simulink model "WindTurbine_System"  (R2023b)
settings: Solver=FixedStepAuto  StartTime=0.0  StopTime=24  FixedStep=1e-6  MaxStep=1e-6  RelTol=1e-3
values from neighbouring files (symbols this model uses):
  c1 = 0.22    [SystemParams.m]    (also in WindTurbineScript.m)
  c2 = 116    [SystemParams.m]    (also in WindTurbineScript.m)
  c3 = 0.4    [SystemParams.m]    (also in WindTurbineScript.m)
  c5 = 5    [SystemParams.m]    (also in WindTurbineScript.m)
  c6 = 12.5    [SystemParams.m]    (also in WindTurbineScript.m)
  C_boost = 50e-6    (= 5e-05)    [SystemParams.m]
  C_buck = 5e-6    (= 5e-06)    [SystemParams.m]
  C_rectifier = 1e-3    (= 0.001)    [SystemParams.m]
  Cp_sys = (Nr_cells_parallel * Cp_cell) / Nr_cells_series    [SystemParams.m]    (also in baterie.m)
  J = 0.8e-3    (= 0.0008)    [SystemParams.m]
  Ke = 0.175    [SystemParams.m]
  L_boost = 200e-6    (= 0.0002)    [SystemParams.m]
  L_buck = 300e-6    (= 0.0003)    [SystemParams.m]
  lambda_opt = 6.33    [SystemParams.m]    (also in WindTurbineScript.m)
  Ld = 1.53e-3    (= 0.00153)    [SystemParams.m]
  Lq = 1.53e-3    (= 0.00153)    [SystemParams.m]
  n1 = 15    [SystemParams.m]
  n2 = 1000    [SystemParams.m]
  omega_r = lambda_opt * wind_speed / R    (= 15.192)    [SystemParams.m]    (also in WindTurbineScript.m = omega_r_values(i))
  p = 4    [SystemParams.m]
  P_buck_v = 1.0e+03 * [0.01, 0.0427, 0.0854, 0.1282, 0.1709, 0.2136, 0.2563, 0.2990, 0.3418, 0.3845, 0.4272,                        0.4699, 0.5126, 0.5554, 0.5981, 0.6408, 0.6835, 0.7262, 0.7690, 0.8117, 0.8544,                        0.8971, 0.9398, 0.9826, 1.0253, 1.0680, 1.1107, 1.1534, 1.1962, 1.2389, 1.2816,                        1.3243, 1.3670, 1.4098, 1.4525, 1.4952, 1.5379, 1.5806, 1.6234, 1.6661, 1. ...(+623 chars)    [SystemParams.m]
  P_rec_v = 1.0e+03 * [0.01, 0.0432, 0.0864, 0.1296, 0.1727, 0.2159, 0.2591, 0.3023, 0.3455, 0.3887, 0.4319,                      0.4750, 0.5182, 0.5614, 0.6046, 0.6478, 0.6910, 0.7342, 0.7773, 0.8205, 0.8637,                      0.9069, 0.9501, 0.9933, 1.0365, 1.0796, 1.1228, 1.1660, 1.2092, 1.2524, 1.2956,                      1.3388, 1.3820, 1.4251, 1.4683, 1.5115, 1.5547, 1.5979, 1.6411, 1.6843, 1.7274,  ...(+605 chars)    [SystemParams.m]
  R = 5    [SystemParams.m]    (also in WindTurbineScript.m)
  R_buck_load_v = [230.4000, 53.9326, 26.9663, 17.9775, 13.4831, 10.7865, 8.9888, 7.7047, 6.7416, 5.9925, 5.3933,                   4.9030, 4.4944, 4.1487, 3.8523, 3.5955, 3.3708, 3.1725, 2.9963, 2.8386, 2.6966, 2.5682,                   2.4515, 2.3449, 2.2472, 2.1573, 2.0743, 1.9975, 1.9262, 1.8597, 1.7978, 1.7398, 1.6854,                   1.6343, 1.5863, 1.5409, 1.4981, 1.4576, 1.4193, 1.3829, 1.3483, 1.3154, 1. ...(+577 chars)    [SystemParams.m]
  R_rec_load_v = 1.0e+03 * [4.8400, 1.1204, 0.5602, 0.3735, 0.2803, 0.2242, 0.1868, 0.1601, 0.1401, 0.1245, 0.1121,                            0.1019, 0.0934, 0.0862, 0.0801, 0.0747, 0.0700, 0.0659, 0.0623, 0.0590, 0.0560, 0.0534,                            0.0509, 0.0487, 0.0467, 0.0448, 0.0431, 0.0415, 0.0400, 0.0386, 0.0374, 0.0362, 0.0350,                            0.0340, 0.0330, 0.0320, 0.0311, 0.0303, 0.02 ...(+634 chars)    [SystemParams.m]
  ro = 1.225    [SystemParams.m]    (also in WindTurbineScript.m)
  Rp_sys = (Nr_cells_series * Rp_cell) / Nr_cells_parallel    [SystemParams.m]    (also in baterie.m)
  Rs = 2.875    [SystemParams.m]    (also in VOC_1C_3pulse_14rest.mat = 0.09415625)
  Rs_sys = (Nr_cells_series * Rs_cell) / Nr_cells_parallel    [SystemParams.m]    (also in baterie.m)
  State_Of_Charge = 65    [SystemParams.m]
libraries: simulink x4, slpidlib x2, SignalEditorBlockLib x1
(part 2 of 2)

== stateflow chart WindTurbine_System/System Control ==
  state No_Wind_Power
    state Battery_Discharge
      entry, during:
      Boost_Control = 1;
      Battery_Control = 1;
      exit:
      Boost_Control = 0;
      Battery_Control = 0;
    state System_Off
      entry, during:
      Battery_Control = 1;
      Boost_Control = 0;
      Buck_Control = 0;
      WindTurbine_Control = 0;
    state Battery_Maintanance
      entry, during:
      Battery_Control = 0;
      Boost_Control = 0;
    (default) -> No_Wind_Power.System_Off
    No_Wind_Power.System_Off -> No_Wind_Power.Battery_Discharge [order 1] : [P_retea > 0 && SOC > 20]
    No_Wind_Power.Battery_Discharge -> No_Wind_Power.System_Off [order 2] : [P_retea == 0]
    No_Wind_Power.Battery_Maintanance -> No_Wind_Power.System_Off : [P_retea == 0]
    No_Wind_Power.System_Off -> No_Wind_Power.Battery_Maintanance [order 2] : [P_retea > 0 && SOC <= 20]
    No_Wind_Power.Battery_Discharge -> No_Wind_Power.Battery_Maintanance [order 1] : [P_retea > 0 && SOC <= 20]
  state Optimal_Wind_Power_Production
    state Battery_Maintanance
      entry, during:
      Battery_Control = 0;
      Buck_Control = 0;
      Boost_Control = 0;
    state Charge_Battery
      entry, during:
      Buck_Control = 1;
      Battery_Control = 1;
      exit:
      Buck_Control = 0;
      Battery_Control = 0;
    state Discharge_Battery
      entry, during:
      Boost_Control = 1;
      Battery_Control = 1;
      exit:
      Boost_Control = 0;
      Battery_Control = 0;
    (default) -> Optimal_Wind_Power_Production.Battery_Maintanance : {WindTurbine_Control = 1}
    Optimal_Wind_Power_Production.Battery_Maintanance -> Optimal_Wind_Power_Production.Charge_Battery [order 1] : [I_dcLink > 0 && SOC <= 80] {Boost_Control = 1;}
    Optimal_Wind_Power_Production.Charge_Battery -> Optimal_Wind_Power_Production.Battery_Maintanance [order 1] : [I_dcLink > 0 && SOC > 80]
    Optimal_Wind_Power_Production.Battery_Maintanance -> Optimal_Wind_Power_Production.Discharge_Battery [order 2] : [I_dcLink < 0 && SOC > 20]
    Optimal_Wind_Power_Production.Discharge_Battery -> Optimal_Wind_Power_Production.Battery_Maintanance [order 1] : [I_dcLink < 0 && SOC <= 20]
    Optimal_Wind_Power_Production.Charge_Battery -> Optimal_Wind_Power_Production.Discharge_Battery [order 2] : [I_dcLink < 0 && SOC <= 80]{Buck_Control = 1}
    Optimal_Wind_Power_Production.Discharge_Battery -> Optimal_Wind_Power_Production.Charge_Battery [order 2] : [I_dcLink > 0 && SOC <= 20 || I_dcLink > 0 && SOC <= 80]
  state High_Wind_Shutdown
    state System_Off
      entry, during:
      WindTurbine_Control = 0;
      Battery_Control = 0;
      Boost_Control = 0;
      Buck_Control = 0;
    state Battery_Discharge
      entry, during:
      Boost_Control = 1;
      Battery_Control = 1;
      exit:
      Boost_Control = 0;
      Battery_Control = 0;
    state Battery_Maintanance
      entry, during:
      Battery_Control = 0;
      Boost_Control = 0;
    (default) -> High_Wind_Shutdown.System_Off : {WindTurbine_Control = 0;}
    High_Wind_Shutdown.System_Off -> High_Wind_Shutdown.Battery_Discharge : [P_retea > 0 && SOC > 20]
    High_Wind_Shutdown.Battery_Maintanance -> High_Wind_Shutdown.System_Off : [P_retea < 0]
    High_Wind_Shutdown.Battery_Discharge -> High_Wind_Shutdown.Battery_Maintanance : [P_retea > 0 && SOC <= 20]
  state Power_Limitation
    state Battery_Maintanance
      entry, during:
      Battery_Control = 0;
      Buck_Control = 0;
      Boost_Control = 0;
    state Charge_Battery
      entry, during:
      Buck_Control = 1;
      Battery_Control = 1;
      exit:
      Buck_Control = 0;
      Battery_Control = 0;
    state Discharge_Battery
      entry, during:
      Boost_Control = 1;
      Battery_Control = 1;
      exit:
      Boost_Control = 0;
      Battery_Control = 0;
    (default) -> Power_Limitation.Battery_Maintanance : {WindTurbine_Control = 1}
    Power_Limitation.Battery_Maintanance -> Power_Limitation.Charge_Battery [order 1] : [I_dcLink > 0 && SOC <= 80]
    Power_Limitation.Charge_Battery -> Power_Limitation.Battery_Maintanance [order 1] : [I_dcLink > 0 && SOC > 80]
    Power_Limitation.Battery_Maintanance -> Power_Limitation.Discharge_Battery [order 2] : [I_dcLink < 0 && SOC > 20]
    Power_Limitation.Discharge_Battery -> Power_Limitation.Battery_Maintanance [order 1] : [I_dcLink < 0 && SOC <= 20]
    Power_Limitation.Discharge_Battery -> Power_Limitation.Charge_Battery [order 2] : [I_dcLink > 0 && SOC <= 20 || I_dcLink > 0 && SOC <= 80]
    Power_Limitation.Charge_Battery -> Power_Limitation.Discharge_Battery [order 2] : [I_dcLink < 0 && SOC <= 80]
  (default) -> No_Wind_Power : {V_cut_in = 7;
      | V_Pwr_Limit = 13;
      | V_cut_out = 20;
      | Battery_Control = 1;
      | }
  No_Wind_Power -> Optimal_Wind_Power_Production : [Wind_speed >= V_cut_in && Wind_speed < V_Pwr_Limit]
  Optimal_Wind_Power_Production -> No_Wind_Power [order 1] : [Wind_speed < V_cut_in]
  Power_Limitation -> Optimal_Wind_Power_Production [order 1] : [Wind_speed < V_Pwr_Limit ]
  Optimal_Wind_Power_Production -> Power_Limitation [order 2] : [Wind_speed >= V_Pwr_Limit && Wind_speed < V_cut_out]
  High_Wind_Shutdown -> No_Wind_Power : [Wind_speed < V_cut_out]
  Power_Limitation -> High_Wind_Shutdown [order 2] : [Wind_speed >= V_cut_out]
  data: Wind_speed input; P_retea input; I_dcLink input; SOC input; Battery_Control output; Boost_Control output; V_Pwr_Limit local; V_cut_in local; V_cut_out local; Buck_Control output; WindTurbine_Control output

== matlab function WindTurbine_System/WTxPMSG/MATLAB Function4 ==
  data: Id input; Ia output; Iq input; theta input; Ib output; Ic output
function [Ia, Ib, Ic] = Inverse_ClarkePark_Current(Id, Iq, theta)

    if isempty(theta)
        theta = 0;
    end

    Ialpha = Id .* cos(theta) - Iq .* sin(theta);
    Ibeta = Id .* sin(theta) + Iq .* cos(theta);

    Ia = Ialpha;
    Ib = Ialpha * (-1)/2 + Ibeta * sqrt(3)/2;
    Ic = Ialpha * (-1)/2 - Ibeta * sqrt(3)/2;


end

== matlab function WindTurbine_System/WTxPMSG/Permanent Magnet Synchronous Generator/MATLAB Function1 ==
  data: Vd input; Va output; Vq input; theta input; Vb output; Vc output
function [Va, Vb, Vc] = Inverse_ClarkePark_Voltage(Vd, Vq, theta)

    if isempty(theta)
        theta = 0;
    end

    Valpha = Vd .* cos(theta) - Vq .* sin(theta);
    Vbeta = Vd .* sin(theta) + Vq .* cos(theta);

    Va = Valpha;
    Vb = Valpha * (-1)/2 + Vbeta * sqrt(3)/2;
    Vc = Valpha * (-1)/2 - Vbeta * sqrt(3)/2;



end

== matlab function WindTurbine_System/WTxPMSG/Permanent Magnet Synchronous Generator/MATLAB Function3 ==
  data: Va input; Vd output; Vb input; Vc input; theta input; Vq output
function [Vd, Vq] = ClarkePark(Va, Vb, Vc, theta)

    if isempty(theta)
        theta = 0;
    end
    
    Valpha = 2/3 * (Va - 0.5 * Vb - 0.5 * Vc);
    Vbeta = 2/3 * (sqrt(3)/2 * Vb - sqrt(3)/2 * Vc);

    Vd = Valpha .* cos(theta) + Vbeta .* sin(theta);
    Vq = -Valpha .* sin(theta) + Vbeta .* cos(theta);

end

== matlab function WindTurbine_System/WTxPMSG/Permanent Magnet Synchronous Generator/MATLAB Function4 ==
  data: Id input; Ia output; Iq input; theta input; Ib output; Ic output
function [Ia, Ib, Ic] = Inverse_ClarkePark_Current(Id, Iq, theta)

    if isempty(theta)
        theta = 0;
    end

    Ialpha = Id .* cos(theta) - Iq .* sin(theta);
    Ibeta = Id .* sin(theta) + Iq .* cos(theta);

    Ia = Ialpha;
    Ib = Ialpha * (-1)/2 + Ibeta * sqrt(3)/2;
    Ic = Ialpha * (-1)/2 - Ibeta * sqrt(3)/2;


end
